simulink model "PID_emulation_be_awu"  (R2022b)
settings: Solver=ode45  StartTime=0.0  StopTime=20  RelTol=1e-3
undefined symbols (not defined in the file): degs2rpm, der, DiscIntNeverNeededParam, drv, gbox, mld, mot, pidz, rads2rpm, rpm2degs, sens, simul, T, Ts
libraries: simulink x3
settings Model: Creator=emanuelevitetta  LastModifiedBy=david

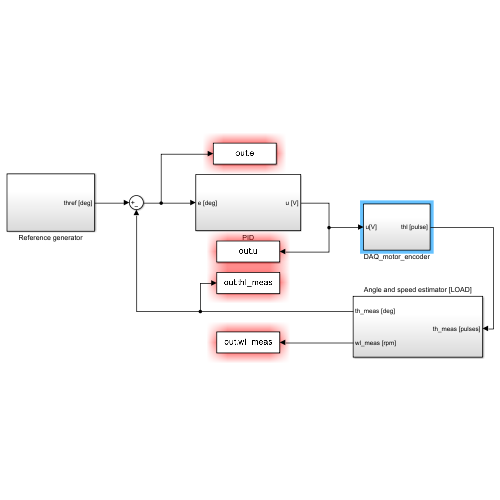
[thumbnail: Simulink's stored preview of the top-level diagram]
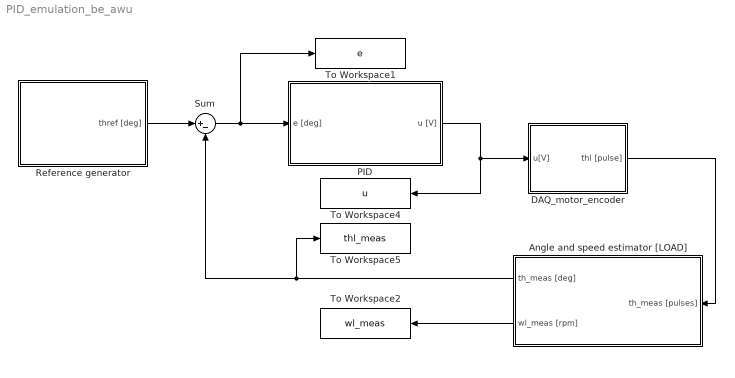
== system PID_emulation_be_awu ==
  Angle and speed estimator [LOAD] : Subsystem
  DAQ_motor_encoder : Subsystem
  PID : Subsystem
  Reference generator : Subsystem
  Sum : Sum  Inputs=|+-
  To Workspace1 : ToWorkspace  VariableName=e  SaveFormat=Structure With Time  SampleTime=Ts
  To Workspace2 : ToWorkspace  VariableName=wl_meas  SaveFormat=Structure With Time  SampleTime=Ts
  To Workspace4 : ToWorkspace  VariableName=u  SaveFormat=Structure With Time  SampleTime=Ts
  To Workspace5 : ToWorkspace  VariableName=thl_meas  SaveFormat=Structure With Time  SampleTime=Ts
  wires:
  PID/1(u [V]) -> DAQ_motor_encoder/1(u[V]), To Workspace4/1
  Sum/1 -> To Workspace1/1, PID/1(e [deg])
  Reference generator/1(thref [deg]) -> Sum/1
  DAQ_motor_encoder/1(thl [pulse]) -> Angle and speed estimator [LOAD]/1(th_meas [pulses])
  Angle and speed estimator [LOAD]/1(th_meas [deg]) -> Sum/2, To Workspace5/1
  Angle and speed estimator [LOAD]/2(wl_meas [rpm]) -> To Workspace2/1

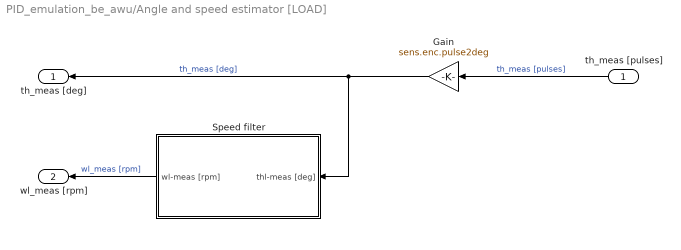
== system PID_emulation_be_awu/Angle and speed estimator [LOAD] ==
  th_meas [pulses] : Inport
  Gain : Gain  Gain=sens.enc.pulse2deg
  Speed filter : Subsystem
  th_meas [deg] : Outport
  wl_meas [rpm] : Outport  Port=2
  wires:
  Speed filter/1(wl-meas [rpm]) -> wl_meas [rpm]/1  "wl_meas [rpm]"
  th_meas [pulses]/1 -> Gain/1  "th_meas [pulses]"
  Gain/1 -> Speed filter/1(thl-meas [deg]), th_meas [deg]/1  "th_meas [deg]"

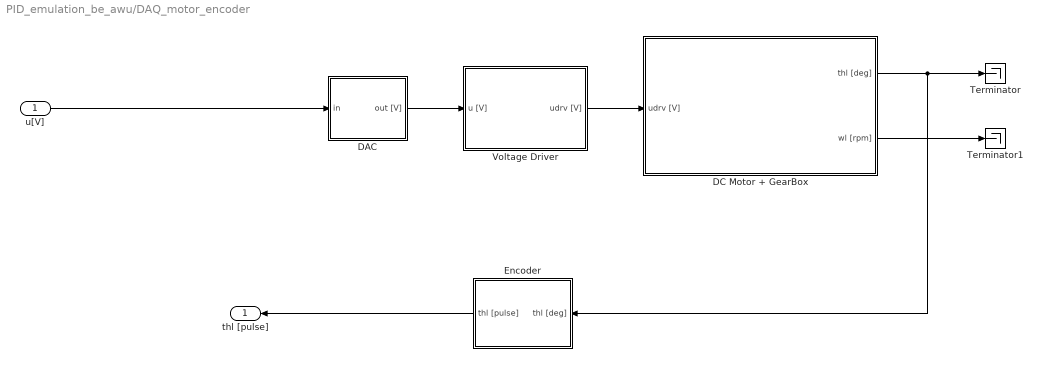
== system PID_emulation_be_awu/DAQ_motor_encoder ==
  u[V] : Inport
  DAC : Subsystem
  DC Motor + GearBox : Subsystem
  Encoder : Subsystem
  Terminator : Terminator
  Terminator1 : Terminator
  Voltage Driver : Subsystem
  thl [pulse] : Outport
  wires:
  DC Motor + GearBox/1(thl [deg]) -> Encoder/1(thl [deg]), Terminator/1
  DC Motor + GearBox/2(wl [rpm]) -> Terminator1/1
  Voltage Driver/1(udrv [V]) -> DC Motor + GearBox/1(udrv [V])
  u[V]/1 -> DAC/1(in)
  DAC/1(out [V]) -> Voltage Driver/1(u [V])
  Encoder/1(thl [pulse]) -> thl [pulse]/1

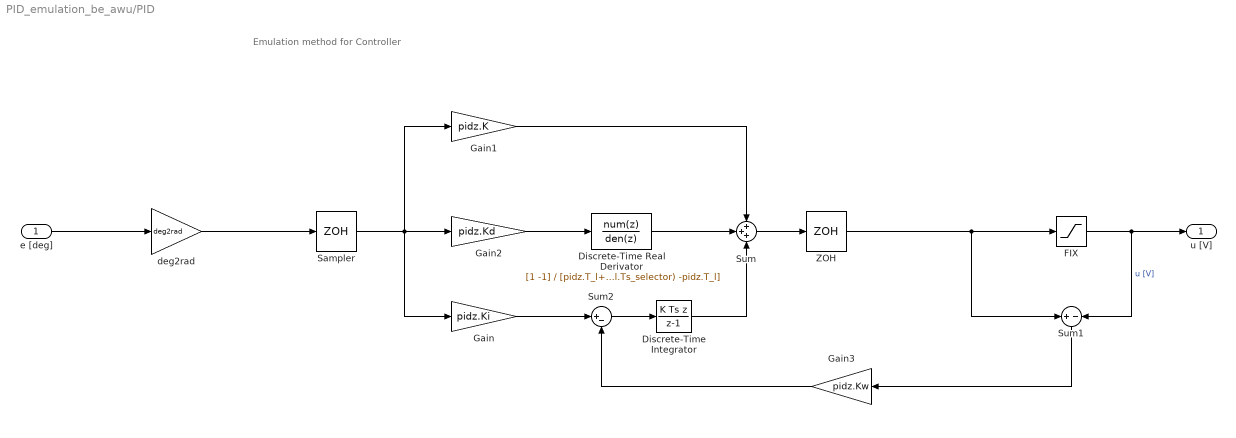
== system PID_emulation_be_awu/PID ==
  note: Emulation method for Controller
  e [deg] : Inport
  Discrete-Time Integrator : DiscreteIntegrator  IntegratorMethod=Integration: Backward Euler  SampleTime=T(simul.Ts_selector)  ICPrevOutput=DiscIntNeverNeededParam  ICPrevScaledInput=DiscIntNeverNeededParam
  "Discrete-Time Real Derivator " : DiscreteTransferFcn  Numerator=[1 -1]  Denominator=[pidz.T_l+T(simul.Ts_selector) -pidz.T_l]  SampleTime=T(simul.Ts_selector)
  "FIX " : Saturate  UpperLimit=10  LowerLimit=-10
  Gain : Gain  Gain=pidz.Ki
  Gain1 : Gain  Gain=pidz.K
  Gain2 : Gain  Gain=pidz.Kd
  Gain3 : Gain  Gain=pidz.Kw
  Sampler : ZeroOrderHold  SampleTime=T(simul.Ts_selector)
  Sum : Sum  Inputs=+++
  Sum1 : Sum  Inputs=+|-
  Sum2 : Sum  Inputs=|+-
  ZOH : ZeroOrderHold  SampleTime=T(simul.Ts_selector)
  deg2rad : Gain  Gain=deg2rad
  u [V] : Outport
  wires:
  e [deg]/1 -> deg2rad/1
  "FIX "/1 -> Sum1/2, u [V]/1  "u [V]"
  deg2rad/1 -> Sampler/1
  ZOH/1 -> Sum1/1, "FIX "/1
  Gain2/1 -> "Discrete-Time Real Derivator "/1
  Sampler/1 -> Gain2/1, Gain1/1, Gain/1
  Gain1/1 -> Sum/1
  Sum/1 -> ZOH/1
  "Discrete-Time Real Derivator "/1 -> Sum/2
  Discrete-Time Integrator/1 -> Sum/3
  Gain/1 -> Sum2/1
  Sum2/1 -> Discrete-Time Integrator/1
  Sum1/1 -> Gain3/1
  Gain3/1 -> Sum2/2

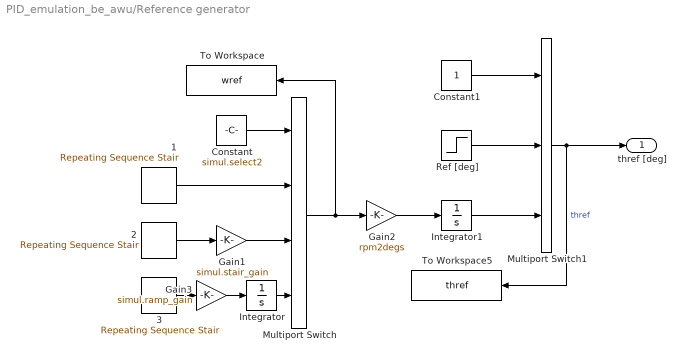
== system PID_emulation_be_awu/Reference generator ==
  1 : simulink/Sources/Repeating Sequence Stair  OutValues=[250 -250].'  tsamp=1  OutMin=[]  OutMax=[]  OutDataTypeStr=double  OutputDataTypeScalingMode=double  OutDataType=fixdt(0,8)  ConRadixGroup=Best Precision: Vector-wise  OutScaling=2^-12
  2 : simulink/Sources/Repeating Sequence Stair  OutValues=[50 100 150 200 250 300 350 400 450 450].'  tsamp=5  OutMin=[]  OutMax=[]  OutDataTypeStr=double  OutputDataTypeScalingMode=double  OutDataType=fixdt(0,8)  ConRadixGroup=Best Precision: Vector-wise  OutScaling=2^-12
  3 : simulink/Sources/Repeating Sequence Stair  OutValues=[450 -450].'  tsamp=1  OutMin=[]  OutMax=[]  OutDataTypeStr=double  OutputDataTypeScalingMode=double  OutDataType=fixdt(0,8)  ConRadixGroup=Best Precision: Vector-wise  OutScaling=2^-12
  Constant : Constant  Value=simul.select2
  Constant1 : Constant
  Gain1 : Gain  Gain=simul.stair_gain
  Gain2 : Gain  Gain=rpm2degs
  Gain3 : Gain  Gain=simul.ramp_gain
  Integrator : Integrator
  Integrator1 : Integrator
  Multiport Switch : MultiPortSwitch  SaturateOnIntegerOverflow=off  InputSameDT=off
  Multiport Switch1 : MultiPortSwitch  Inputs=2  SaturateOnIntegerOverflow=off  InputSameDT=off
  Ref [deg] : Step  After=simul.stepdeg
  To Workspace : ToWorkspace  VariableName=wref  SaveFormat=Timeseries  SampleTime=Ts
  To Workspace5 : ToWorkspace  VariableName=thref  SaveFormat=Structure With Time  SampleTime=Ts
  thref [deg] : Outport
  wires:
  Integrator1/1 -> Multiport Switch1/3
  Constant/1 -> Multiport Switch/1
  Gain1/1 -> Multiport Switch/3
  2/1 -> Gain1/1
  Gain2/1 -> Integrator1/1
  Integrator/1 -> Multiport Switch/4
  1/1 -> Multiport Switch/2
  3/1 -> Gain3/1
  Gain3/1 -> Integrator/1
  Ref [deg]/1 -> Multiport Switch1/2
  Constant1/1 -> Multiport Switch1/1
  Multiport Switch1/1 -> thref [deg]/1, To Workspace5/1  "thref"
  Multiport Switch/1 -> Gain2/1, To Workspace/1

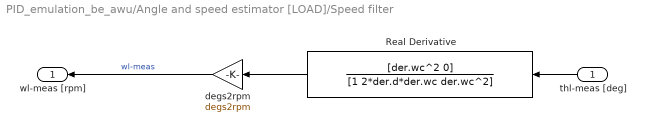
== system PID_emulation_be_awu/Angle and speed estimator [LOAD]/Speed filter ==
  thl-meas [deg] : Inport
  Real Derivative : TransferFcn  Numerator=[der.wc^2 0]  Denominator=[1 2*der.d*der.wc der.wc^2]
  degs2rpm : Gain  Gain=degs2rpm
  wl-meas [rpm] : Outport
  wires:
  thl-meas [deg]/1 -> Real Derivative/1
  degs2rpm/1 -> wl-meas [rpm]/1  "wl-meas"
  Real Derivative/1 -> degs2rpm/1

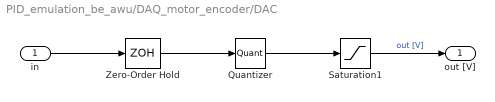
== system PID_emulation_be_awu/DAQ_motor_encoder/DAC ==
  in : Inport
  Quantizer : Quantizer  QuantizationInterval=daq.dac.q
  Saturation1 : Saturate  UpperLimit=10  LowerLimit=-10
  Zero-Order Hold : ZeroOrderHold  SampleTime=Ts
  out [V] : Outport
  wires:
  Saturation1/1 -> out [V]/1  "out [V]"
  in/1 -> Zero-Order Hold/1
  Zero-Order Hold/1 -> Quantizer/1
  Quantizer/1 -> Saturation1/1

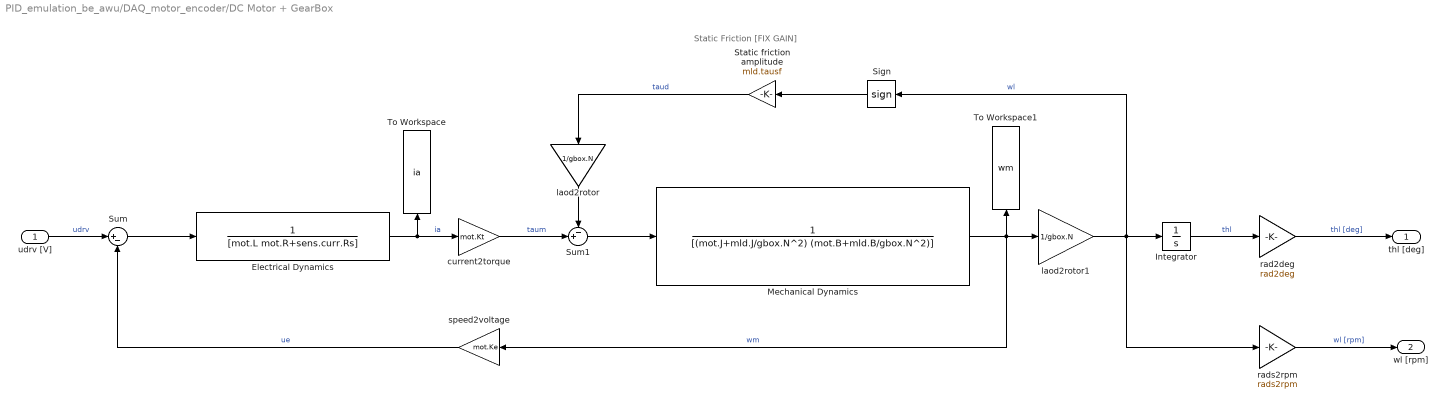
== system PID_emulation_be_awu/DAQ_motor_encoder/DC Motor + GearBox ==
  note: Static Friction [FIX GAIN]
  udrv [V] : Inport
  Electrical Dynamics : TransferFcn  Denominator=[mot.L mot.R+sens.curr.Rs]
  Integrator : Integrator
  Mechanical Dynamics : TransferFcn  Denominator=[(mot.J+mld.J/gbox.N^2) (mot.B+mld.B/gbox.N^2)]
  Sign : Signum  ZeroCross=off
  Static friction amplitude : Gain  Gain=mld.tausf
  Sum : Sum  Inputs=|+-
  Sum1 : Sum  Inputs=-+|
  To Workspace : ToWorkspace  VariableName=ia  SaveFormat=Timeseries  SampleTime=-1
  To Workspace1 : ToWorkspace  VariableName=wm  SaveFormat=Timeseries  SampleTime=-1
  current2torque : Gain  Gain=mot.Kt
  laod2rotor : Gain  Gain=1/gbox.N
  laod2rotor1 : Gain  Gain=1/gbox.N
  rad2deg : Gain  Gain=rad2deg
  rads2rpm : Gain  Gain=rads2rpm
  speed2voltage : Gain  Gain=mot.Ke
  thl [deg] : Outport
  wl [rpm] : Outport  Port=2
  wires:
  rads2rpm/1 -> wl [rpm]/1  "wl [rpm]"
  Sign/1 -> Static friction amplitude/1
  Electrical Dynamics/1 -> To Workspace/1, current2torque/1  "ia"
  Sum1/1 -> Mechanical Dynamics/1
  laod2rotor1/1 -> rads2rpm/1, Sign/1, Integrator/1  "wl"
  rad2deg/1 -> thl [deg]/1  "thl [deg]"
  laod2rotor/1 -> Sum1/1
  udrv [V]/1 -> Sum/1  "udrv"
  current2torque/1 -> Sum1/2  "taum"
  Static friction amplitude/1 -> laod2rotor/1  "taud"
  speed2voltage/1 -> Sum/2  "ue"
  Integrator/1 -> rad2deg/1  "thl"
  Sum/1 -> Electrical Dynamics/1
  Mechanical Dynamics/1 -> laod2rotor1/1, To Workspace1/1, speed2voltage/1  "wm"

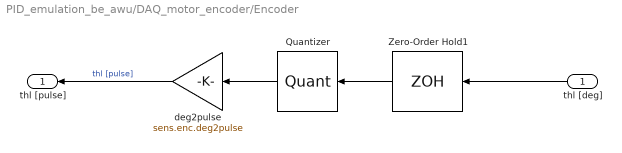
== system PID_emulation_be_awu/DAQ_motor_encoder/Encoder ==
  thl [deg] : Inport
  Quantizer : Quantizer  QuantizationInterval=sens.enc.pulse2deg
  Zero-Order Hold1 : ZeroOrderHold  SampleTime=Ts
  deg2pulse : Gain  Gain=sens.enc.deg2pulse
  thl [pulse] : Outport
  wires:
  thl [deg]/1 -> Zero-Order Hold1/1
  Zero-Order Hold1/1 -> Quantizer/1
  deg2pulse/1 -> thl [pulse]/1  "thl [pulse]"
  Quantizer/1 -> deg2pulse/1

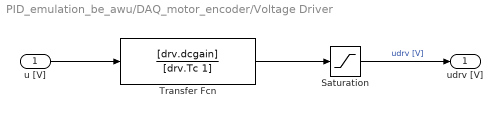
== system PID_emulation_be_awu/DAQ_motor_encoder/Voltage Driver ==
  u [V] : Inport
  Saturation : Saturate  UpperLimit=12  LowerLimit=-12
  Transfer Fcn : TransferFcn  Numerator=[drv.dcgain]  Denominator=[drv.Tc 1]
  udrv [V] : Outport
  wires:
  Saturation/1 -> udrv [V]/1  "udrv [V]"
  u [V]/1 -> Transfer Fcn/1
  Transfer Fcn/1 -> Saturation/1
